simulink model "plant_test"  (R2023b)
settings: Solver=VariableStepAuto  StartTime=0.0  StopTime=t_end  RelTol=1e-3
values from neighbouring files (symbols this model uses):
  dt = (2*pi)/(100*w)    [plot_bode.m]    (also in plot_impulse.m = 0.0001; plot_initial.m = 0.0001)
  sysc = plant_sysc(param,option)    [plot_bode.m]    (also in plot_impulse.m; plot_initial.m)
  w = w_vec(i)    [plot_bode.m]
  x0 = 0    [plot_bode.m]    (also in plot_impulse.m; plot_initial.m = 50000)
undefined symbols (not defined in the file or in its folder): ue, xe
libraries: fl_lib x10, nesl_utility x4
(part 1 of 3)
settings Model: Creator=MPC5  LastModifiedBy=MPC5

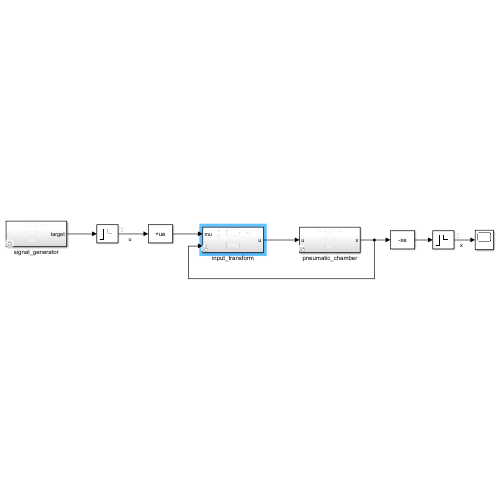
[thumbnail: Simulink's stored preview of the top-level diagram]
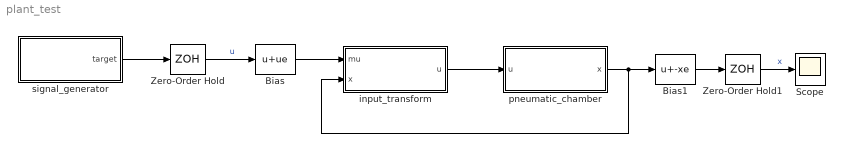
== system plant_test ==
  Bias : Bias  Bias=ue  SaturateOnIntegerOverflow=off
  Bias1 : Bias  Bias=-xe  SaturateOnIntegerOverflow=off
  Scope : Scope
  Zero-Order Hold : ZeroOrderHold  SampleTime=dt
  Zero-Order Hold1 : ZeroOrderHold  SampleTime=dt
  input_transform : Subsystem  Variant=on
  pneumatic_chamber : Subsystem  Variant=on
  signal_generator : Subsystem  Variant=on
  wires:
  Zero-Order Hold/1 -> Bias/1  "u"
  Bias/1 -> input_transform/1(mu)
  pneumatic_chamber/1(x) -> input_transform/2(x), Bias1/1
  Zero-Order Hold1/1 -> Scope/1  "x"
  signal_generator/1(target) -> Zero-Order Hold/1
  Bias1/1 -> Zero-Order Hold1/1
  input_transform/1(u) -> pneumatic_chamber/1(u)

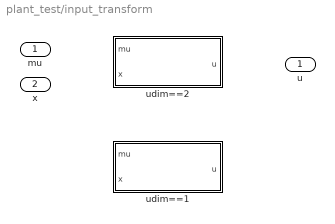
== system plant_test/input_transform ==
  mu : Inport
  x : Inport  Port=2
  udim==1 : Subsystem  VariantControl="plant_model_type == \"sysc\""
  udim==2 : Subsystem  VariantControl="plant_model_type == \"simscape\" || plant_model_type == \"ode\""
  u : Outport

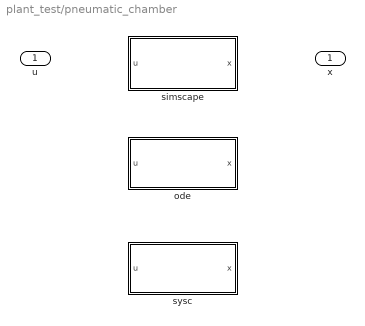
== system plant_test/pneumatic_chamber ==
  u : Inport
  ode : Subsystem  VariantControl="plant_model_type==\"ode\""
  simscape : Subsystem  VariantControl="plant_model_type==\"simscape\""
  sysc : Subsystem  VariantControl="plant_model_type==\"sysc\""
  x : Outport

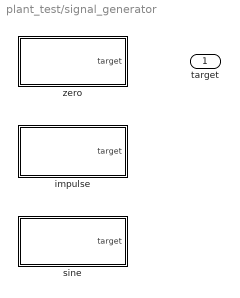
== system plant_test/signal_generator ==
  impulse : Subsystem  VariantControl="input_signal_type==\"impulse\""
  sine : Subsystem  VariantControl="input_signal_type==\"sine\""
  zero : Subsystem  VariantControl="input_signal_type==\"zero\""
  target : Outport

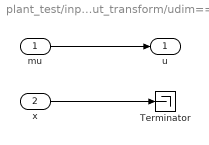
== system plant_test/input_transform/udim==1 ==
  mu : Inport
  x : Inport  Port=2
  Terminator : Terminator
  u : Outport
  wires:
  mu/1 -> u/1
  x/1 -> Terminator/1

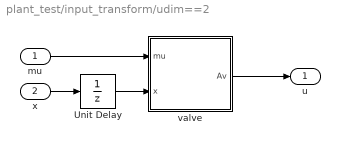
== system plant_test/input_transform/udim==2 ==
  mu : Inport
  x : Inport  Port=2
  Unit Delay : UnitDelay  InitialCondition=x0  SampleTime=-1  HasFrameUpgradeWarning=on
  valve : MATLAB Function  TreatAsAtomicUnit=on
  u : Outport
  wires:
  valve/1(Av) -> u/1
  mu/1 -> valve/1(mu)
  x/1 -> Unit Delay/1
  Unit Delay/1 -> valve/2(x)

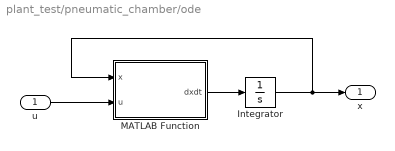
== system plant_test/pneumatic_chamber/ode ==
  u : Inport
  Integrator : Integrator  InitialCondition=x0
  MATLAB Function : MATLAB Function  TreatAsAtomicUnit=on
  x : Outport
  wires:
  MATLAB Function/1(dxdt) -> Integrator/1
  u/1 -> MATLAB Function/2(u)
  Integrator/1 -> x/1, MATLAB Function/1(x)
